simulink model "permutematrix_ref"  (Simulink 4.00)
settings: Solver=FixedStepDiscrete  StartTime=0.0  StopTime=10.0  RelTol=1e-3
PostLoadFcn:
  | set_param(gcs,'SimulationCommand','Update')
libraries: dspsrcs3 x2, dspmtrx3 x2
settings Model: RequirementInfo=9  Creator=ckamachi  LastModifiedBy=ckamachi  LimitDataPoints=off  ExtModeTrigMode=oneshot  ExtModeArmWhenConnect=off  BlockReductionOpt=off

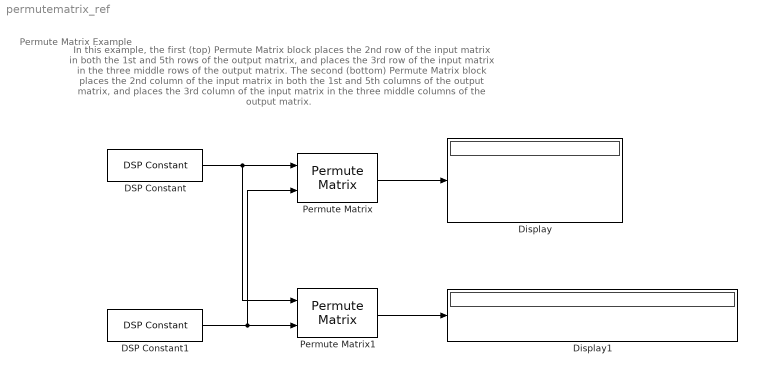
== system permutematrix_ref ==
  note: Permute Matrix Example
  note: In this example, the first (top) Permute Matrix block places the 2nd row of the input matrix in both the
      | 1st and 5th rows of the output matrix, and places the 3rd row of the input matrix in the three middle
      | rows of the output matrix. The second (bottom) Permute Matrix block places the 2nd column of the
      | input matrix in both the 1st and 5th columns of the output matrix, and places the 3rd column of the
      | input matrix in the three middle columns of the output matrix.
  DSP Constant : dspsrcs3/DSP Constant  Value=[1 2 3;4 5 6;7 8 9]  InterpretAs1D=off  SampleMode=Discrete  Ts=1  FramebasedOutput=off
  DSP Constant1 : dspsrcs3/DSP Constant  Value=[2 3 3 3 2]  InterpretAs1D=off  SampleMode=Discrete  Ts=1  FramebasedOutput=off
  Display : Display
      settings: Format=short
  Display1 : Display
      settings: Format=short
  Permute Matrix : dspmtrx3/Permute Matrix  mode=Rows  errmode=Clip Index  checkDims=off
  Permute Matrix1 : dspmtrx3/Permute Matrix  mode=Columns  errmode=Clip Index  checkDims=off
  wires:
  DSP Constant/1 -> Permute Matrix/1, Permute Matrix1/1
  Permute Matrix/1 -> Display/1
  Permute Matrix1/1 -> Display1/1
  DSP Constant1/1 -> Permute Matrix1/2, Permute Matrix/2
